simulink model "ex4_1"  (R2018b)
settings: Solver=VariableStepAuto  StartTime=0.0  StopTime=200.0  RelTol=1e-3
values from neighbouring files (symbols this model uses):
  a1 = 1    [ex4_script.m]
  a2 = 1    [ex4_script.m]
  g = 10    [ex4_script.m]
  k = 5    [ex4_script.m]
  m = 70    [ex4_script.m]
settings Model: Creator=HYJ  LastModifiedBy=HYJ
settings SFSimCC: SimUseLocalCustomCode=off
settings RTWCC: RTWUseLocalCustomCode=off

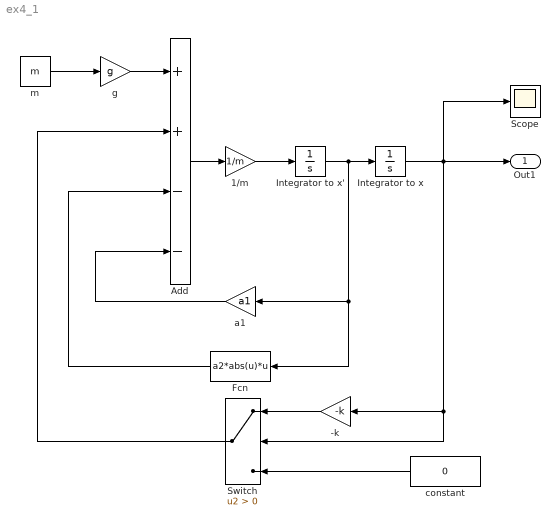
== system ex4_1 ==
  " Integrator to x" : Integrator
  -k : Gain  Gain=-k
  1/m : Gain  Gain=1/m
  Add : Sum  Inputs=++--
  Fcn : Fcn  Expr=a2*abs(u)*u
  Integrator to x' : Integrator
  Scope : Scope
  Switch : Switch  Criteria=u2 > Threshold
  a1 : Gain  Gain=a1
  constant : Constant  Value=0
  g : Gain  Gain=g
  m : Constant  Value=m
  Out1 : Outport
  wires:
  Integrator to x'/1 -> Fcn/1, a1/1, " Integrator to x"/1
  " Integrator to x"/1 -> Switch/2, -k/1, Scope/1, Out1/1
  Add/1 -> 1/m/1
  1/m/1 -> Integrator to x'/1
  a1/1 -> Add/4
  Fcn/1 -> Add/3
  m/1 -> g/1
  g/1 -> Add/1
  constant/1 -> Switch/3
  -k/1 -> Switch/1
  Switch/1 -> Add/2
